simulink model "session 8 page 44"  (R2021b)
settings: Solver=VariableStepAuto  StartTime=0.0  StopTime=10.0  RelTol=1e-3
settings Model: Creator=Pixle  LastModifiedBy=Pixle

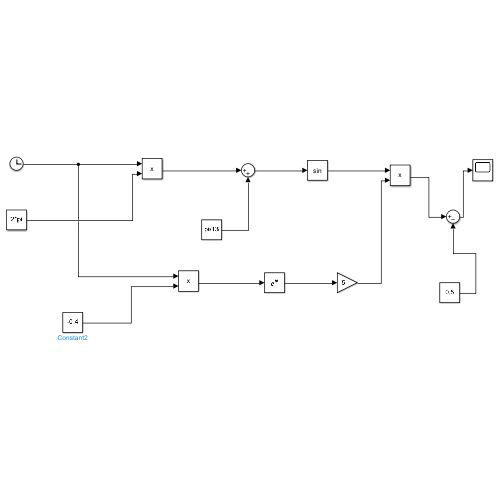
[thumbnail: Simulink's stored preview of the top-level diagram]
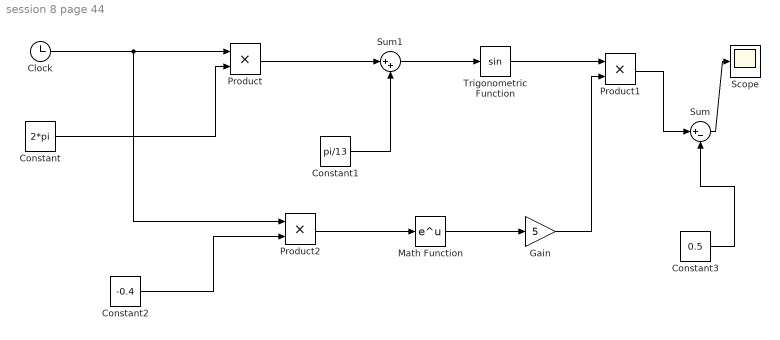
== system session 8 page 44 ==
  Clock : Clock
  Constant : Constant  Value=2*pi
  Constant1 : Constant  Value=pi/13
  Constant2 : Constant  Value=-0.4
  Constant3 : Constant  Value=0.5
  Gain : Gain  Gain=5
  Math Function : Math  SaturateOnIntegerOverflow=on
  Product : Product
  Product1 : Product
  Product2 : Product
  Scope : Scope
  Sum : Sum  Inputs=|+-
  Sum1 : Sum  Inputs=|++
  Trigonometric Function : Trigonometry
  wires:
  Clock/1 -> Product2/1, Product/1
  Constant/1 -> Product/2
  Constant1/1 -> Sum1/2
  Product/1 -> Sum1/1
  Constant2/1 -> Product2/2
  Sum1/1 -> Trigonometric Function/1
  Trigonometric Function/1 -> Product1/1
  Product2/1 -> Math Function/1
  Math Function/1 -> Gain/1
  Gain/1 -> Product1/2
  Constant3/1 -> Sum/2
  Product1/1 -> Sum/1
  Sum/1 -> Scope/1
